simulink model "BrakeSystem_Hydraulics"  (R2021b)
settings: Solver=VariableStepAuto  StartTime=0.0  StopTime=20  RelTol=1e-3
undefined symbols (not defined in the file): Caliper_F_Damp, fcdb
libraries: fl_lib x75, sdl_lib x3, nesl_utility x3, simulink x1, sh_lib x1
settings Model: Creator=pgzar  LastModifiedBy=pgzar

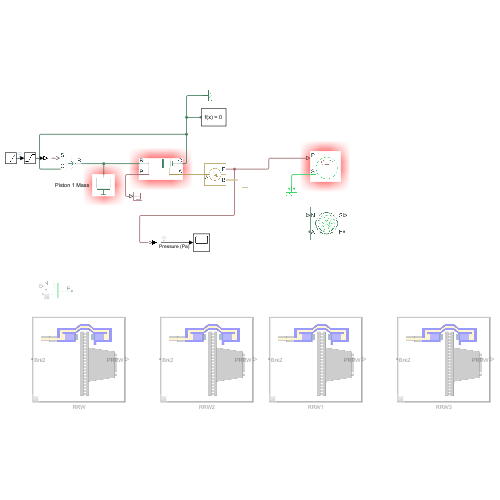
[thumbnail: Simulink's stored preview of the top-level diagram]
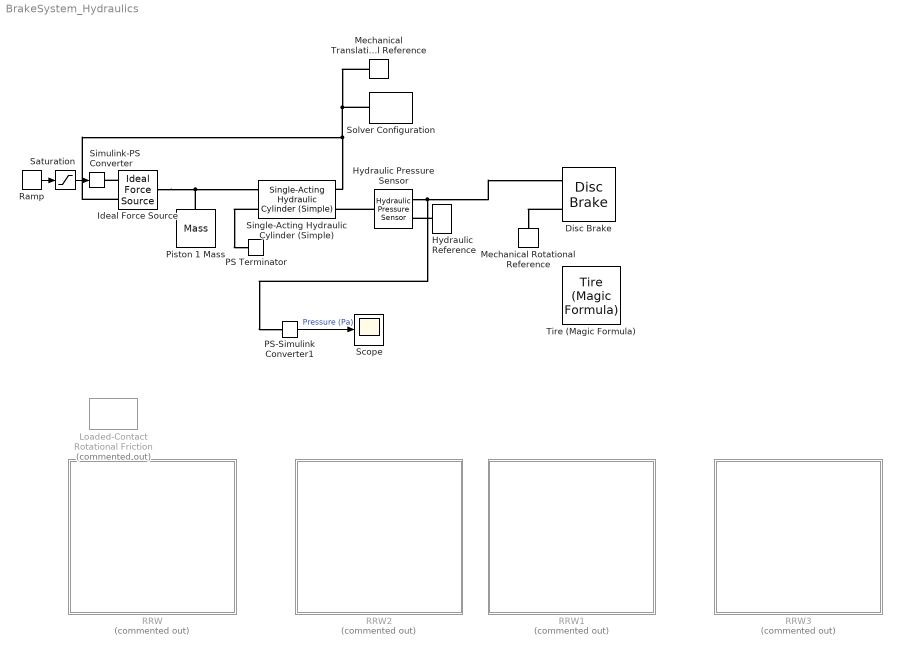
== system BrakeSystem_Hydraulics ==
  Disc Brake : sdl_lib/Brakes & Detents/Rotational/Disc Brake  r_mean=Caliper_PadMeanRadius mm  bore=Caliper_F_PistonDiameter mm  n_pads=2  thermal_port=simscape.enum.thermaleffects.omit  mu_static=Pad_StaticFirctionCoef  mu_coulomb=Pad_ClulombFrictionCoef  temperature_TLU=[280, 300, 320] K  mu_static_TLU=[.9, .8, .7]  mu_coulomb_TLU=[.8, .7, .6]  brkwy_vel=Pad_BrakeawayFrictionVel rad/s  visc_coef=0 N*m/(rad/s)  enable_faults=simscape.enum.onoff.off  faulted_pressure=0 bar  external_fault=simscape.enum.onoff.off  temporal_fault=simscape.enum.onoff.off  fault_time=5 s  report_fault=simscape.enum.assert.action.none  thermal_mass=50 kJ/K  temperature_specify=off  temperature_priority=High  temperature=300 K  temperature_nominal_specify=off  temperature_nominal_unit=K  temperature_nominal_value=1
      settings: SourceProductBaseCode=LD
  Hydraulic Pressure Sensor : fl_lib/Hydraulic/Hydraulic Sensors/Hydraulic Pressure Sensor
  Hydraulic Reference : fl_lib/Hydraulic/Hydraulic Elements/Hydraulic Reference
  Ideal Force Source : fl_lib/Mechanical/Mechanical Sources/Ideal Force Source
  Loaded-Contact Rotational Friction : sdl_lib/Brakes & Detents/Rotational/Loaded-Contact Rotational Friction  Commented=on  geometry_model=sdl.enum.friction_geometry.radius  r_eff=130 mm  d_o=150 mm  d_i=100 mm  friction_model=sdl.enum.friction_model_TLU_thermal.fixed  mu_w_vector=[0, 100, 1000] rad/s  temperature_TLU=[280, 300, 320] K  mu_static=0.35  mu_static_vector=[.4, .38, .36]  mu_coulomb=0.3  mu_coulomb_vector=[.3, .22, .19]  mu_coulomb_temp_vector=[.3, .28, .25]  mu_coulomb_matrix=[.34, .32, .3; .3, .28, .25; .25, .2, .15]  mu_interp_method=simscape.enum.interpolation.linear  mu_extrap_method=simscape.enum.extrapolation.linear  w_tol=0.001 rad/s  force_min=1 N  mu_visc=0 N*m*s/rad  initial_state_locked=sdl.enum.initial_lock.unlocked  enable_faults=simscape.enum.onoff.off  fault_type=sdl.enum.clutchFault.lock  external_fault=simscape.enum.onoff.off  temporal_fault=simscape.enum.onoff.off  fault_time=5 s  report_fault=simscape.enum.assert.action.none  thermal_mass=50 kJ/K  T_init=300 K
      settings: SourceProductBaseCode=LD  InternalSimscapePortConfiguration="{\"Bottom\":[],\"Left\":[{\"id\":\"N\",\"label\":\"N\",\"type\":\"input\"},{\"id\":\"B\",\"label\":\"B\",\"type\":\"foundation.mechanical.rotational.rotational\"}],\"Right\":[{\"id\":\"F\",\"label\":\"F\",\"type\":\"foundation.mechanical.rotational.rotational\"}],\"Top\":[]}"
  Mechanical Rotational Reference : fl_lib/Mechanical/Rotational Elements/Mechanical Rotational Reference
  Mechanical Translational Reference : fl_lib/Mechanical/Translational Elements/Mechanical Translational Reference
  PS Terminator : fl_lib/Physical Signals/Sinks/PS Terminator
  PS-Simulink Converter1 : nesl_utility/PS-Simulink Converter  PhysicalDomain=network_engine_domain  SubClassName=ps_output  LeftPortType=input  RightPortType=output  PseudoPeriodic=off  Frequencies=[]  Unit=inherit  AffineConversion=off
      settings: SourceProductBaseCode=PW,SS
  Piston 1 Mass : fl_lib/Mechanical/Translational Elements/Mass  mass=MC_F_PistonMass kg  num_ports=foundation.enum.numPorts2.one  v_specify=off  v_priority=High  v=0 m/s  v_nominal_specify=off  v_nominal_unit=m/s  v_nominal_value=1  f_specify=off  f_priority=None  f=0 N  f_nominal_specify=off  f_nominal_unit=N  f_nominal_value=1
  RRW : Subsystem  Commented=on
      mask Display:
      | image('sscfluids_braking_caliper_disk_brake.png');
      | port_label('LConn',1,'Brk2')
      | port_label('RConn',1,'PRRW')
  RRW1 : Subsystem  Commented=on
      mask Display:
      | image('sscfluids_braking_caliper_disk_brake.png');
      | port_label('LConn',1,'Brk2')
      | port_label('RConn',1,'PRRW')
  RRW2 : Subsystem  Commented=on
      mask Display:
      | image('sscfluids_braking_caliper_disk_brake.png');
      | port_label('LConn',1,'Brk2')
      | port_label('RConn',1,'PRRW')
  RRW3 : Subsystem  Commented=on
      mask Display:
      | image('sscfluids_braking_caliper_disk_brake.png');
      | port_label('LConn',1,'Brk2')
      | port_label('RConn',1,'PRRW')
  Ramp : simulink/Sources/Ramp  slope=10000000  start=0.1  InitialOutput=0
  Saturation : Saturate  UpperLimit=1000000  LowerLimit=0
  Scope : Scope
  Simulink-PS Converter : nesl_utility/Simulink-PS Converter  PhysicalDomain=network_engine_domain  SubClassName=ps_input  LeftPortType=input  RightPortType=output  PseudoPeriodic=off  Frequencies=[]  NoiseDistribution=none  NoiseParameters=[]  Unit=N  AffineConversion=off  FilteringAndDerivatives=provide  SimscapeFilterOrder=1  InputFilterTimeConstant=0.001  UdotUserProvided=0
      settings: SourceProductBaseCode=PW,SS
  Single-Acting Hydraulic Cylinder (Simple) : sh_lib/Hydraulic Cylinders/Single-Acting Hydraulic Cylinder (Simple)  area=MC_F_PistonArea m^2  stroke=MC_F_PistonStroke m  init_pos=0 m  penetr_coeff=1e12 N*s/m^2  or=2
      settings: SourceProductBaseCode=SH  InternalSimscapePortConfiguration="{\"Bottom\":[],\"Left\":[{\"id\":\"C\",\"label\":\"C\",\"type\":\"foundation.mechanical.translational.translational\"},{\"id\":\"A\",\"label\":\"A\",\"type\":\"foundation.hydraulic.hydraulic\"}],\"Right\":[{\"id\":\"R\",\"label\":\"R\",\"type\":\"foundation.mechanical.translational.translational\"},{\"id\":\"P\",\"label\":\"P\",\"type\":\"output\"}],\"Top\":[]}"
  Solver Configuration : nesl_utility/Solver Configuration  PhysicalDomain=network_engine_domain  SubClassName=solver  LeftPortType=input  RightPortType=generic  Tones=[]  Harmonics=[]  SimulateNoise=off  Profile=off  UseLocalSampling=off  EnableSwitchedLinearOptims=on  FrequencyDomain=off  UseCCode=off  RelTol=0.001  AbsTol=1e-06  MinStep=1e-09  ToWorkspace=off  RevertToSquareIcSolve=off  NumHomotopyIterations=100  PhasorMode=off  PhasorModeNumHarmonics=1  DoDC=off  ResidualTolerance=1e-09  UseLocalSolver=off  LocalSolverChoice=NE_BACKWARD_EULER_ADVANCER  LocalSolverSampleTime=0.001  DoFixedCost=off  MaxNonlinIter=3  MaxModeIter=2  ComputeImpulses=off  ImpulseIterations=2  LinearAlgebra=auto  EquationFormulation=NE_TIME_EF  DelaysMemoryBudget=1024  AutomaticFiltering=on  FilteringTimeConstant=0.001  PartitionStorageMethod=AS_NEEDED  PartitionMemoryBudget=1024  PartitionMethod=ROBUST
      settings: SourceProductBaseCode=PW,SS
  Tire (Magic Formula) : sdl_lib/Tires & Vehicles/Tire (Magic Formula)  parameterization=sdl.enum.magic_tire_model.peak  F_z1=3000 N  F_x1=3500 N  kappa1=10  B_m=10  C_m=1.9  D_m=1  E_m=0.97  fz0=4000 N  p_Cx=1.685  p_Dx=[1.21, -.037]  p_Ex=[.344, .095, -.02, 0]  p_Kx=[21.51, -.163, .245]  p_Hx=[-.002, .002]  p_Vx=[0, 0]  r_e=0.3 m  model_compliance=sdl.enum.compliance.off  stiffness=1e6 N/m  damping=1000 N*s/m  model_inertia=sdl.enum.model_inertia.off  inertia=1 kg*m^2  initial_velocity=0 rad/s  model_resistance=simscape.enum.onoff.off  resistance_model=sdl.enum.rollingResistanceParameterization.constant  coeff=0.015  p_tire=250e3 Pa  alpha=-0.003  beta=0.97  coeff_a=84e-4  coeff_b=6.2e-4 s/m  coeff_c=1.6e-4 s^2/m^2  v_thr=0.001 m/s  v_tr_thr=0.1 m/s
  wires:
  Ramp/1 -> Saturation/1
  PS-Simulink Converter1/1 -> Scope/1  "Pressure (Pa)"
  Saturation/1 -> Simulink-PS Converter/1
  connections:
  Piston 1 Mass/LConn1 -- Ideal Force Source/LConn1 -- Single-Acting Hydraulic Cylinder (Simple)/RConn1
  Mechanical Translational Reference/LConn1 -- Ideal Force Source/RConn2 -- Single-Acting Hydraulic Cylinder (Simple)/LConn1 -- Solver Configuration/RConn1
  Ideal Force Source/RConn1 -- Simulink-PS Converter/RConn1
  Hydraulic Pressure Sensor/RConn2 -- PS-Simulink Converter1/LConn1 -- Disc Brake/LConn1
  Hydraulic Pressure Sensor/LConn1 -- Single-Acting Hydraulic Cylinder (Simple)/LConn2
  Hydraulic Reference/LConn1 -- Hydraulic Pressure Sensor/RConn1
  Disc Brake/LConn2 -- Mechanical Rotational Reference/LConn1
  Single-Acting Hydraulic Cylinder (Simple)/RConn2 -- PS Terminator/LConn1

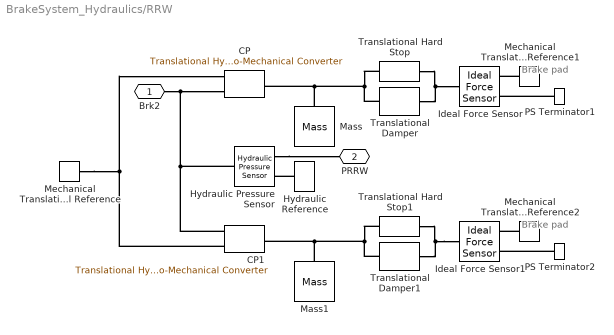
== system BrakeSystem_Hydraulics/RRW ==
  note: Brake pad
  note: Brake pad
  CP : fl_lib/Hydraulic/Hydraulic Elements/Translational Hydro-Mechanical Converter  area=Caliper_F_PistonArea m^2  or=1  compressibility=simscape.enum.onoff.on  displacement_spec=foundation.enum.DisplacementSpec.Calculate  init_pos=0 m  V_dead=Caliper_F_DeadVolume m^3  k_sh=1.4  initial_pressure=Caliper_F_InitialPressure Pa
      settings: SourceProductBaseCode=SS  InternalSimscapePortConfiguration="{\"Bottom\":[],\"Left\":[{\"id\":\"C\",\"label\":\"C\",\"type\":\"foundation.mechanical.translational.translational\"},{\"id\":\"A\",\"label\":\"A\",\"type\":\"foundation.hydraulic.hydraulic\"}],\"Right\":[{\"id\":\"R\",\"label\":\"R\",\"type\":\"foundation.mechanical.translational.translational\"}],\"Top\":[]}"
  CP1 : fl_lib/Hydraulic/Hydraulic Elements/Translational Hydro-Mechanical Converter  area=Caliper_F_PistonArea m^2  or=1  compressibility=simscape.enum.onoff.on  displacement_spec=foundation.enum.DisplacementSpec.Calculate  init_pos=0 m  V_dead=Caliper_F_DeadVolume m^3  k_sh=1.4  initial_pressure=Caliper_F_InitialPressure Pa
      settings: SourceProductBaseCode=SS  InternalSimscapePortConfiguration="{\"Bottom\":[],\"Left\":[{\"id\":\"C\",\"label\":\"C\",\"type\":\"foundation.mechanical.translational.translational\"},{\"id\":\"A\",\"label\":\"A\",\"type\":\"foundation.hydraulic.hydraulic\"}],\"Right\":[{\"id\":\"R\",\"label\":\"R\",\"type\":\"foundation.mechanical.translational.translational\"}],\"Top\":[]}"
  Hydraulic Pressure Sensor : fl_lib/Hydraulic/Hydraulic Sensors/Hydraulic Pressure Sensor
  Hydraulic Reference : fl_lib/Hydraulic/Hydraulic Elements/Hydraulic Reference
  Ideal Force Sensor : fl_lib/Mechanical/Mechanical Sensors/Ideal Force Sensor
  Ideal Force Sensor1 : fl_lib/Mechanical/Mechanical Sensors/Ideal Force Sensor
  Mass : fl_lib/Mechanical/Translational Elements/Mass  mass=Caliper_F_PistonMass kg  num_ports=foundation.enum.numPorts2.one  v_specify=off  v_priority=High  v=0 m/s  v_nominal_specify=off  v_nominal_unit=m/s  v_nominal_value=1  f_specify=off  f_priority=None  f=0 N  f_nominal_specify=off  f_nominal_unit=N  f_nominal_value=1
  Mass1 : fl_lib/Mechanical/Translational Elements/Mass  mass=Caliper_F_PistonMass kg  num_ports=foundation.enum.numPorts2.one  v_specify=off  v_priority=High  v=0 m/s  v_nominal_specify=off  v_nominal_unit=m/s  v_nominal_value=1  f_specify=off  f_priority=None  f=0 N  f_nominal_specify=off  f_nominal_unit=N  f_nominal_value=1
  Mechanical Translational Reference : fl_lib/Mechanical/Translational Elements/Mechanical Translational Reference
  Mechanical Translational Reference1 : fl_lib/Mechanical/Translational Elements/Mechanical Translational Reference
  Mechanical Translational Reference2 : fl_lib/Mechanical/Translational Elements/Mechanical Translational Reference
  PS Terminator1 : fl_lib/Physical Signals/Sinks/PS Terminator
  PS Terminator2 : fl_lib/Physical Signals/Sinks/PS Terminator
  Translational Damper : fl_lib/Mechanical/Translational Elements/Translational Damper  D=Caliper_F_Damp N/(m/s)  v_specify=off  v_priority=None  v=0 m/s  v_nominal_specify=off  v_nominal_unit=m/s  v_nominal_value=1  f_specify=off  f_priority=None  f=0 N  f_nominal_specify=off  f_nominal_unit=N  f_nominal_value=1
  Translational Damper1 : fl_lib/Mechanical/Translational Elements/Translational Damper  D=Caliper_F_Damp N/(m/s)  v_specify=off  v_priority=None  v=0 m/s  v_nominal_specify=off  v_nominal_unit=m/s  v_nominal_value=1  f_specify=off  f_priority=None  f=0 N  f_nominal_specify=off  f_nominal_unit=N  f_nominal_value=1
  Translational Hard Stop : fl_lib/Mechanical/Translational Elements/Translational Hard Stop  upper_bnd=Caliper_F_RunClear m  lower_bnd=0 m  stiff_up=Caliper_F_ComplianceR N/m  stiff_low=Caliper_F_HSS N/m  D_up=Caliper_F_Damp N/(m/s)  D_low=Caliper_F_HSD N/(m/s)  model=simscape.enum.hardstop.smooth  transition=0.1 mm  v_specify=off  v_priority=None  v=0 m/s  v_nominal_specify=off  v_nominal_unit=m/s  v_nominal_value=1  f_specify=off  f_priority=None  f=0 N  f_nominal_specify=off  f_nominal_unit=N  f_nominal_value=1  x_specify=off  x_priority=High  x=0 m  x_nominal_specify=off  x_nominal_unit=m  x_nominal_value=1
  Translational Hard Stop1 : fl_lib/Mechanical/Translational Elements/Translational Hard Stop  upper_bnd=Caliper_F_RunClear m  lower_bnd=0 m  stiff_up=Caliper_F_ComplianceR N/m  stiff_low=Caliper_F_HSS N/m  D_up=Caliper_F_Damp N/(m/s)  D_low=Caliper_F_HSD N/(m/s)  model=simscape.enum.hardstop.smooth  transition=0.1 mm  v_specify=off  v_priority=None  v=0 m/s  v_nominal_specify=off  v_nominal_unit=m/s  v_nominal_value=1  f_specify=off  f_priority=None  f=0 N  f_nominal_specify=off  f_nominal_unit=N  f_nominal_value=1  x_specify=off  x_priority=High  x=0 m  x_nominal_specify=off  x_nominal_unit=m  x_nominal_value=1
  Brk2 : PMIOPort  Side=Left
  PRRW : PMIOPort  Port=2  Side=Right
  connections:
  Mass/LConn1 -- Translational Damper/LConn1 -- Translational Hard Stop/LConn1 -- CP/RConn1
  Translational Hard Stop/RConn1 -- Translational Damper/RConn1 -- Ideal Force Sensor/LConn1
  Mechanical Translational Reference/LConn1 -- CP/LConn1 -- CP1/LConn1
  Hydraulic Pressure Sensor/LConn1 -- Brk2/RConn1 -- CP/LConn2 -- CP1/LConn2
  Hydraulic Pressure Sensor/RConn2 -- PRRW/RConn1
  Hydraulic Reference/LConn1 -- Hydraulic Pressure Sensor/RConn1
  PS Terminator1/LConn1 -- Ideal Force Sensor/RConn2
  Mechanical Translational Reference1/LConn1 -- Ideal Force Sensor/RConn1
  Ideal Force Sensor1/LConn1 -- Translational Hard Stop1/RConn1 -- Translational Damper1/RConn1
  Translational Hard Stop1/LConn1 -- Mass1/LConn1 -- CP1/RConn1 -- Translational Damper1/LConn1
  Mechanical Translational Reference2/LConn1 -- Ideal Force Sensor1/RConn1
  PS Terminator2/LConn1 -- Ideal Force Sensor1/RConn2

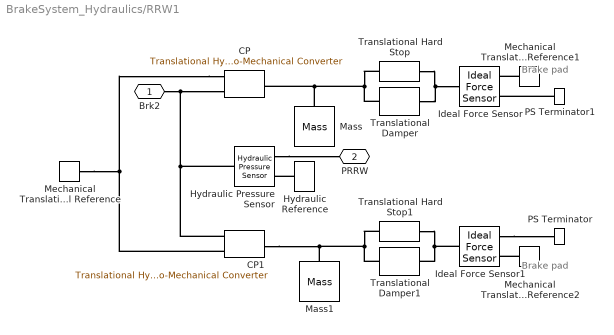
== system BrakeSystem_Hydraulics/RRW1 ==
  note: Brake pad
  note: Brake pad
  CP : fl_lib/Hydraulic/Hydraulic Elements/Translational Hydro-Mechanical Converter  area=fcdb.area m^2  or=1  compressibility=simscape.enum.onoff.on  displacement_spec=foundation.enum.DisplacementSpec.Calculate  init_pos=0 m  V_dead=fcdb.deadV m^3  k_sh=1.4  initial_pressure=tpc.pRes Pa
      settings: SourceProductBaseCode=SS  InternalSimscapePortConfiguration="{\"Bottom\":[],\"Left\":[{\"id\":\"C\",\"label\":\"C\",\"type\":\"foundation.mechanical.translational.translational\"},{\"id\":\"A\",\"label\":\"A\",\"type\":\"foundation.hydraulic.hydraulic\"}],\"Right\":[{\"id\":\"R\",\"label\":\"R\",\"type\":\"foundation.mechanical.translational.translational\"}],\"Top\":[]}"
  CP1 : fl_lib/Hydraulic/Hydraulic Elements/Translational Hydro-Mechanical Converter  area=fcdb.area m^2  or=1  compressibility=simscape.enum.onoff.on  displacement_spec=foundation.enum.DisplacementSpec.Calculate  init_pos=0 m  V_dead=fcdb.deadV m^3  k_sh=1.4  initial_pressure=tpc.pRes Pa
      settings: SourceProductBaseCode=SS  InternalSimscapePortConfiguration="{\"Bottom\":[],\"Left\":[{\"id\":\"C\",\"label\":\"C\",\"type\":\"foundation.mechanical.translational.translational\"},{\"id\":\"A\",\"label\":\"A\",\"type\":\"foundation.hydraulic.hydraulic\"}],\"Right\":[{\"id\":\"R\",\"label\":\"R\",\"type\":\"foundation.mechanical.translational.translational\"}],\"Top\":[]}"
  Hydraulic Pressure Sensor : fl_lib/Hydraulic/Hydraulic Sensors/Hydraulic Pressure Sensor
  Hydraulic Reference : fl_lib/Hydraulic/Hydraulic Elements/Hydraulic Reference
  Ideal Force Sensor : fl_lib/Mechanical/Mechanical Sensors/Ideal Force Sensor
  Ideal Force Sensor1 : fl_lib/Mechanical/Mechanical Sensors/Ideal Force Sensor
  Mass : fl_lib/Mechanical/Translational Elements/Mass  mass=fcdb.mass kg  num_ports=foundation.enum.numPorts2.one  v_specify=off  v_priority=High  v=0 m/s  v_nominal_specify=off  v_nominal_unit=m/s  v_nominal_value=1  f_specify=off  f_priority=None  f=0 N  f_nominal_specify=off  f_nominal_unit=N  f_nominal_value=1
  Mass1 : fl_lib/Mechanical/Translational Elements/Mass  mass=fcdb.mass kg  num_ports=foundation.enum.numPorts2.one  v_specify=off  v_priority=High  v=0 m/s  v_nominal_specify=off  v_nominal_unit=m/s  v_nominal_value=1  f_specify=off  f_priority=None  f=0 N  f_nominal_specify=off  f_nominal_unit=N  f_nominal_value=1
  Mechanical Translational Reference : fl_lib/Mechanical/Translational Elements/Mechanical Translational Reference
  Mechanical Translational Reference1 : fl_lib/Mechanical/Translational Elements/Mechanical Translational Reference
  Mechanical Translational Reference2 : fl_lib/Mechanical/Translational Elements/Mechanical Translational Reference
  PS Terminator : fl_lib/Physical Signals/Sinks/PS Terminator
  PS Terminator1 : fl_lib/Physical Signals/Sinks/PS Terminator
  Translational Damper : fl_lib/Mechanical/Translational Elements/Translational Damper  D=fcdb.damp N/(m/s)  v_specify=off  v_priority=None  v=0 m/s  v_nominal_specify=off  v_nominal_unit=m/s  v_nominal_value=1  f_specify=off  f_priority=None  f=0 N  f_nominal_specify=off  f_nominal_unit=N  f_nominal_value=1
  Translational Damper1 : fl_lib/Mechanical/Translational Elements/Translational Damper  D=fcdb.damp N/(m/s)  v_specify=off  v_priority=None  v=0 m/s  v_nominal_specify=off  v_nominal_unit=m/s  v_nominal_value=1  f_specify=off  f_priority=None  f=0 N  f_nominal_specify=off  f_nominal_unit=N  f_nominal_value=1
  Translational Hard Stop : fl_lib/Mechanical/Translational Elements/Translational Hard Stop  upper_bnd=fcdb.runClear m  lower_bnd=0 m  stiff_up=fcdb.complianceR N/m  stiff_low=fcdb.hss N/m  D_up=fcdb.damp N/(m/s)  D_low=fcdb.hsd N/(m/s)  model=simscape.enum.hardstop.smooth  transition=0.1 mm  v_specify=off  v_priority=None  v=0 m/s  v_nominal_specify=off  v_nominal_unit=m/s  v_nominal_value=1  f_specify=off  f_priority=None  f=0 N  f_nominal_specify=off  f_nominal_unit=N  f_nominal_value=1  x_specify=off  x_priority=High  x=0 m  x_nominal_specify=off  x_nominal_unit=m  x_nominal_value=1
  Translational Hard Stop1 : fl_lib/Mechanical/Translational Elements/Translational Hard Stop  upper_bnd=fcdb.runClear m  lower_bnd=0 m  stiff_up=fcdb.complianceR N/m  stiff_low=fcdb.hss N/m  D_up=fcdb.damp N/(m/s)  D_low=fcdb.hsd N/(m/s)  model=simscape.enum.hardstop.smooth  transition=0.1 mm  v_specify=off  v_priority=None  v=0 m/s  v_nominal_specify=off  v_nominal_unit=m/s  v_nominal_value=1  f_specify=off  f_priority=None  f=0 N  f_nominal_specify=off  f_nominal_unit=N  f_nominal_value=1  x_specify=off  x_priority=High  x=0 m  x_nominal_specify=off  x_nominal_unit=m  x_nominal_value=1
  Brk2 : PMIOPort  Side=Left
  PRRW : PMIOPort  Port=2  Side=Right
  connections:
  Mass/LConn1 -- Translational Damper/LConn1 -- Translational Hard Stop/LConn1 -- CP/RConn1
  Translational Hard Stop/RConn1 -- Translational Damper/RConn1 -- Ideal Force Sensor/LConn1
  CP/LConn1 -- CP1/LConn1 -- Mechanical Translational Reference/LConn1
  CP1/LConn2 -- Hydraulic Pressure Sensor/LConn1 -- Brk2/RConn1 -- CP/LConn2
  Translational Damper1/LConn1 -- CP1/RConn1 -- Mass1/LConn1 -- Translational Hard Stop1/LConn1
  Ideal Force Sensor1/LConn1 -- Translational Hard Stop1/RConn1 -- Translational Damper1/RConn1
  Hydraulic Pressure Sensor/RConn2 -- PRRW/RConn1
  Hydraulic Reference/LConn1 -- Hydraulic Pressure Sensor/RConn1
  Ideal Force Sensor1/RConn2 -- PS Terminator/LConn1
  PS Terminator1/LConn1 -- Ideal Force Sensor/RConn2
  Mechanical Translational Reference1/LConn1 -- Ideal Force Sensor/RConn1
  Mechanical Translational Reference2/LConn1 -- Ideal Force Sensor1/RConn1

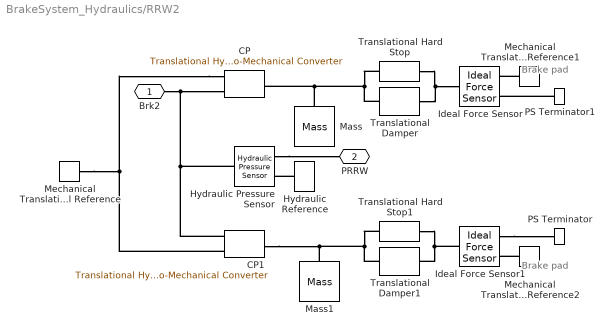
== system BrakeSystem_Hydraulics/RRW2 ==
  note: Brake pad
  note: Brake pad
  CP : fl_lib/Hydraulic/Hydraulic Elements/Translational Hydro-Mechanical Converter  area=fcdb.area m^2  or=1  compressibility=simscape.enum.onoff.on  displacement_spec=foundation.enum.DisplacementSpec.Calculate  init_pos=0 m  V_dead=fcdb.deadV m^3  k_sh=1.4  initial_pressure=tpc.pRes Pa
      settings: SourceProductBaseCode=SS  InternalSimscapePortConfiguration="{\"Bottom\":[],\"Left\":[{\"id\":\"C\",\"label\":\"C\",\"type\":\"foundation.mechanical.translational.translational\"},{\"id\":\"A\",\"label\":\"A\",\"type\":\"foundation.hydraulic.hydraulic\"}],\"Right\":[{\"id\":\"R\",\"label\":\"R\",\"type\":\"foundation.mechanical.translational.translational\"}],\"Top\":[]}"
  CP1 : fl_lib/Hydraulic/Hydraulic Elements/Translational Hydro-Mechanical Converter  area=fcdb.area m^2  or=1  compressibility=simscape.enum.onoff.on  displacement_spec=foundation.enum.DisplacementSpec.Calculate  init_pos=0 m  V_dead=fcdb.deadV m^3  k_sh=1.4  initial_pressure=tpc.pRes Pa
      settings: SourceProductBaseCode=SS  InternalSimscapePortConfiguration="{\"Bottom\":[],\"Left\":[{\"id\":\"C\",\"label\":\"C\",\"type\":\"foundation.mechanical.translational.translational\"},{\"id\":\"A\",\"label\":\"A\",\"type\":\"foundation.hydraulic.hydraulic\"}],\"Right\":[{\"id\":\"R\",\"label\":\"R\",\"type\":\"foundation.mechanical.translational.translational\"}],\"Top\":[]}"
  Hydraulic Pressure Sensor : fl_lib/Hydraulic/Hydraulic Sensors/Hydraulic Pressure Sensor
  Hydraulic Reference : fl_lib/Hydraulic/Hydraulic Elements/Hydraulic Reference
  Ideal Force Sensor : fl_lib/Mechanical/Mechanical Sensors/Ideal Force Sensor
  Ideal Force Sensor1 : fl_lib/Mechanical/Mechanical Sensors/Ideal Force Sensor
  Mass : fl_lib/Mechanical/Translational Elements/Mass  mass=fcdb.mass kg  num_ports=foundation.enum.numPorts2.one  v_specify=off  v_priority=High  v=0 m/s  v_nominal_specify=off  v_nominal_unit=m/s  v_nominal_value=1  f_specify=off  f_priority=None  f=0 N  f_nominal_specify=off  f_nominal_unit=N  f_nominal_value=1
  Mass1 : fl_lib/Mechanical/Translational Elements/Mass  mass=fcdb.mass kg  num_ports=foundation.enum.numPorts2.one  v_specify=off  v_priority=High  v=0 m/s  v_nominal_specify=off  v_nominal_unit=m/s  v_nominal_value=1  f_specify=off  f_priority=None  f=0 N  f_nominal_specify=off  f_nominal_unit=N  f_nominal_value=1
  Mechanical Translational Reference : fl_lib/Mechanical/Translational Elements/Mechanical Translational Reference
  Mechanical Translational Reference1 : fl_lib/Mechanical/Translational Elements/Mechanical Translational Reference
  Mechanical Translational Reference2 : fl_lib/Mechanical/Translational Elements/Mechanical Translational Reference
  PS Terminator : fl_lib/Physical Signals/Sinks/PS Terminator
  PS Terminator1 : fl_lib/Physical Signals/Sinks/PS Terminator
  Translational Damper : fl_lib/Mechanical/Translational Elements/Translational Damper  D=fcdb.damp N/(m/s)  v_specify=off  v_priority=None  v=0 m/s  v_nominal_specify=off  v_nominal_unit=m/s  v_nominal_value=1  f_specify=off  f_priority=None  f=0 N  f_nominal_specify=off  f_nominal_unit=N  f_nominal_value=1
  Translational Damper1 : fl_lib/Mechanical/Translational Elements/Translational Damper  D=fcdb.damp N/(m/s)  v_specify=off  v_priority=None  v=0 m/s  v_nominal_specify=off  v_nominal_unit=m/s  v_nominal_value=1  f_specify=off  f_priority=None  f=0 N  f_nominal_specify=off  f_nominal_unit=N  f_nominal_value=1
  Translational Hard Stop : fl_lib/Mechanical/Translational Elements/Translational Hard Stop  upper_bnd=fcdb.runClear m  lower_bnd=0 m  stiff_up=fcdb.complianceR N/m  stiff_low=fcdb.hss N/m  D_up=fcdb.damp N/(m/s)  D_low=fcdb.hsd N/(m/s)  model=simscape.enum.hardstop.smooth  transition=0.1 mm  v_specify=off  v_priority=None  v=0 m/s  v_nominal_specify=off  v_nominal_unit=m/s  v_nominal_value=1  f_specify=off  f_priority=None  f=0 N  f_nominal_specify=off  f_nominal_unit=N  f_nominal_value=1  x_specify=off  x_priority=High  x=0 m  x_nominal_specify=off  x_nominal_unit=m  x_nominal_value=1
  Translational Hard Stop1 : fl_lib/Mechanical/Translational Elements/Translational Hard Stop  upper_bnd=fcdb.runClear m  lower_bnd=0 m  stiff_up=fcdb.complianceR N/m  stiff_low=fcdb.hss N/m  D_up=fcdb.damp N/(m/s)  D_low=fcdb.hsd N/(m/s)  model=simscape.enum.hardstop.smooth  transition=0.1 mm  v_specify=off  v_priority=None  v=0 m/s  v_nominal_specify=off  v_nominal_unit=m/s  v_nominal_value=1  f_specify=off  f_priority=None  f=0 N  f_nominal_specify=off  f_nominal_unit=N  f_nominal_value=1  x_specify=off  x_priority=High  x=0 m  x_nominal_specify=off  x_nominal_unit=m  x_nominal_value=1
  Brk2 : PMIOPort  Side=Left
  PRRW : PMIOPort  Port=2  Side=Right
  connections:
  Mass/LConn1 -- Translational Damper/LConn1 -- Translational Hard Stop/LConn1 -- CP/RConn1
  Translational Hard Stop/RConn1 -- Translational Damper/RConn1 -- Ideal Force Sensor/LConn1
  CP/LConn1 -- CP1/LConn1 -- Mechanical Translational Reference/LConn1
  CP1/LConn2 -- Hydraulic Pressure Sensor/LConn1 -- Brk2/RConn1 -- CP/LConn2
  Translational Damper1/LConn1 -- CP1/RConn1 -- Mass1/LConn1 -- Translational Hard Stop1/LConn1
  Ideal Force Sensor1/LConn1 -- Translational Hard Stop1/RConn1 -- Translational Damper1/RConn1
  Hydraulic Pressure Sensor/RConn2 -- PRRW/RConn1
  Hydraulic Reference/LConn1 -- Hydraulic Pressure Sensor/RConn1
  Ideal Force Sensor1/RConn2 -- PS Terminator/LConn1
  PS Terminator1/LConn1 -- Ideal Force Sensor/RConn2
  Mechanical Translational Reference1/LConn1 -- Ideal Force Sensor/RConn1
  Mechanical Translational Reference2/LConn1 -- Ideal Force Sensor1/RConn1

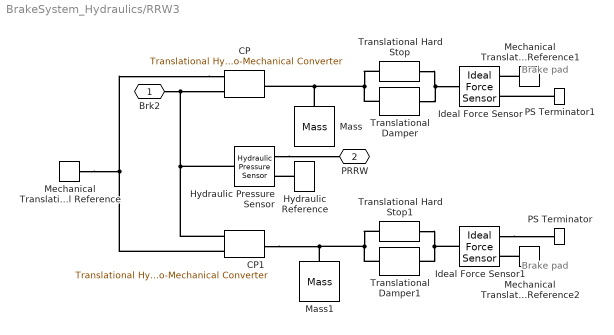
== system BrakeSystem_Hydraulics/RRW3 ==
  note: Brake pad
  note: Brake pad
  CP : fl_lib/Hydraulic/Hydraulic Elements/Translational Hydro-Mechanical Converter  area=fcdb.area m^2  or=1  compressibility=simscape.enum.onoff.on  displacement_spec=foundation.enum.DisplacementSpec.Calculate  init_pos=0 m  V_dead=fcdb.deadV m^3  k_sh=1.4  initial_pressure=tpc.pRes Pa
      settings: SourceProductBaseCode=SS  InternalSimscapePortConfiguration="{\"Bottom\":[],\"Left\":[{\"id\":\"C\",\"label\":\"C\",\"type\":\"foundation.mechanical.translational.translational\"},{\"id\":\"A\",\"label\":\"A\",\"type\":\"foundation.hydraulic.hydraulic\"}],\"Right\":[{\"id\":\"R\",\"label\":\"R\",\"type\":\"foundation.mechanical.translational.translational\"}],\"Top\":[]}"
  CP1 : fl_lib/Hydraulic/Hydraulic Elements/Translational Hydro-Mechanical Converter  area=fcdb.area m^2  or=1  compressibility=simscape.enum.onoff.on  displacement_spec=foundation.enum.DisplacementSpec.Calculate  init_pos=0 m  V_dead=fcdb.deadV m^3  k_sh=1.4  initial_pressure=tpc.pRes Pa
      settings: SourceProductBaseCode=SS  InternalSimscapePortConfiguration="{\"Bottom\":[],\"Left\":[{\"id\":\"C\",\"label\":\"C\",\"type\":\"foundation.mechanical.translational.translational\"},{\"id\":\"A\",\"label\":\"A\",\"type\":\"foundation.hydraulic.hydraulic\"}],\"Right\":[{\"id\":\"R\",\"label\":\"R\",\"type\":\"foundation.mechanical.translational.translational\"}],\"Top\":[]}"
  Hydraulic Pressure Sensor : fl_lib/Hydraulic/Hydraulic Sensors/Hydraulic Pressure Sensor
  Hydraulic Reference : fl_lib/Hydraulic/Hydraulic Elements/Hydraulic Reference
  Ideal Force Sensor : fl_lib/Mechanical/Mechanical Sensors/Ideal Force Sensor
  Ideal Force Sensor1 : fl_lib/Mechanical/Mechanical Sensors/Ideal Force Sensor
  Mass : fl_lib/Mechanical/Translational Elements/Mass  mass=fcdb.mass kg  num_ports=foundation.enum.numPorts2.one  v_specify=off  v_priority=High  v=0 m/s  v_nominal_specify=off  v_nominal_unit=m/s  v_nominal_value=1  f_specify=off  f_priority=None  f=0 N  f_nominal_specify=off  f_nominal_unit=N  f_nominal_value=1
  Mass1 : fl_lib/Mechanical/Translational Elements/Mass  mass=fcdb.mass kg  num_ports=foundation.enum.numPorts2.one  v_specify=off  v_priority=High  v=0 m/s  v_nominal_specify=off  v_nominal_unit=m/s  v_nominal_value=1  f_specify=off  f_priority=None  f=0 N  f_nominal_specify=off  f_nominal_unit=N  f_nominal_value=1
  Mechanical Translational Reference : fl_lib/Mechanical/Translational Elements/Mechanical Translational Reference
  Mechanical Translational Reference1 : fl_lib/Mechanical/Translational Elements/Mechanical Translational Reference
  Mechanical Translational Reference2 : fl_lib/Mechanical/Translational Elements/Mechanical Translational Reference
  PS Terminator : fl_lib/Physical Signals/Sinks/PS Terminator
  PS Terminator1 : fl_lib/Physical Signals/Sinks/PS Terminator
  Translational Damper : fl_lib/Mechanical/Translational Elements/Translational Damper  D=fcdb.damp N/(m/s)  v_specify=off  v_priority=None  v=0 m/s  v_nominal_specify=off  v_nominal_unit=m/s  v_nominal_value=1  f_specify=off  f_priority=None  f=0 N  f_nominal_specify=off  f_nominal_unit=N  f_nominal_value=1
  Translational Damper1 : fl_lib/Mechanical/Translational Elements/Translational Damper  D=fcdb.damp N/(m/s)  v_specify=off  v_priority=None  v=0 m/s  v_nominal_specify=off  v_nominal_unit=m/s  v_nominal_value=1  f_specify=off  f_priority=None  f=0 N  f_nominal_specify=off  f_nominal_unit=N  f_nominal_value=1
  Translational Hard Stop : fl_lib/Mechanical/Translational Elements/Translational Hard Stop  upper_bnd=fcdb.runClear m  lower_bnd=0 m  stiff_up=fcdb.complianceR N/m  stiff_low=fcdb.hss N/m  D_up=fcdb.damp N/(m/s)  D_low=fcdb.hsd N/(m/s)  model=simscape.enum.hardstop.smooth  transition=0.1 mm  v_specify=off  v_priority=None  v=0 m/s  v_nominal_specify=off  v_nominal_unit=m/s  v_nominal_value=1  f_specify=off  f_priority=None  f=0 N  f_nominal_specify=off  f_nominal_unit=N  f_nominal_value=1  x_specify=off  x_priority=High  x=0 m  x_nominal_specify=off  x_nominal_unit=m  x_nominal_value=1
  Translational Hard Stop1 : fl_lib/Mechanical/Translational Elements/Translational Hard Stop  upper_bnd=fcdb.runClear m  lower_bnd=0 m  stiff_up=fcdb.complianceR N/m  stiff_low=fcdb.hss N/m  D_up=fcdb.damp N/(m/s)  D_low=fcdb.hsd N/(m/s)  model=simscape.enum.hardstop.smooth  transition=0.1 mm  v_specify=off  v_priority=None  v=0 m/s  v_nominal_specify=off  v_nominal_unit=m/s  v_nominal_value=1  f_specify=off  f_priority=None  f=0 N  f_nominal_specify=off  f_nominal_unit=N  f_nominal_value=1  x_specify=off  x_priority=High  x=0 m  x_nominal_specify=off  x_nominal_unit=m  x_nominal_value=1
  Brk2 : PMIOPort  Side=Left
  PRRW : PMIOPort  Port=2  Side=Right
  connections:
  Mass/LConn1 -- Translational Damper/LConn1 -- Translational Hard Stop/LConn1 -- CP/RConn1
  Translational Hard Stop/RConn1 -- Translational Damper/RConn1 -- Ideal Force Sensor/LConn1
  CP/LConn1 -- CP1/LConn1 -- Mechanical Translational Reference/LConn1
  CP1/LConn2 -- Hydraulic Pressure Sensor/LConn1 -- Brk2/RConn1 -- CP/LConn2
  Translational Damper1/LConn1 -- CP1/RConn1 -- Mass1/LConn1 -- Translational Hard Stop1/LConn1
  Ideal Force Sensor1/LConn1 -- Translational Hard Stop1/RConn1 -- Translational Damper1/RConn1
  Hydraulic Pressure Sensor/RConn2 -- PRRW/RConn1
  Hydraulic Reference/LConn1 -- Hydraulic Pressure Sensor/RConn1
  Ideal Force Sensor1/RConn2 -- PS Terminator/LConn1
  PS Terminator1/LConn1 -- Ideal Force Sensor/RConn2
  Mechanical Translational Reference1/LConn1 -- Ideal Force Sensor/RConn1
  Mechanical Translational Reference2/LConn1 -- Ideal Force Sensor1/RConn1
